simulink model "All_Car_Models"  (R2018b)
settings: Solver=VariableStepAuto  StartTime=0.0  StopTime=10.0  RelTol=1e-3
values from neighbouring files (symbols this model uses):
  a = 1.25    [SetCoefficients_FC.m]
  amplitude = 0.01    [SetCoefficients_FC.m]
  b = 1.4    [SetCoefficients_FC.m]
  c = 1.3    [SetCoefficients_FC.m]
  csc = 600    [SetCoefficients_FC.m]
  cse = 1200    [SetCoefficients_FC.m]
  d = 1.7    [SetCoefficients_FC.m]
  delay = (a+b)/v    [setSpeed.m]
  Fre_r = Fre*2*pi    [setSpeed.m]
  g = 9.81    [SetCoefficients_FC.m]
  HumpHight = 2    [SetCoefficients_FC.m]
  HumpLegnth = 20    [SetCoefficients_FC.m]
  I = 600    [SetCoefficients_FC.m]
  I_phi = 1000    [SetCoefficients_FC.m]
  I_theta = 600    [SetCoefficients_FC.m]
  ks =     [SetCoefficients.m]    (also in SetCoefficients_FC.m = 20000)
  ksSteel = 6.6e9    (= 6600000000)    [SetCoefficients_FC.m]
  ksstiff = 4e5    (= 400000)    [SetCoefficients_FC.m]
  kt =     [SetCoefficients.m]    (also in SetCoefficients_FC.m = 140000)
  m1 = 250    [SetCoefficients.m]    (also in SetCoefficients_FC.m)
  m2 =     [SetCoefficients.m]    (also in SetCoefficients_FC.m = 20)
  mb = 1000    [SetCoefficients_FC.m]
  mbh = mb/2    (= 500)    [SetCoefficients_FC.m]
  v_hump = v    [setSpeed.m]
  x1 = 0.2    [SetCoefficients_FC.m]
  x2 = 0.25    [SetCoefficients_FC.m]
  xt_Lim = 0.1    [SetCoefficients_FC.m]
(part 2 of 2)

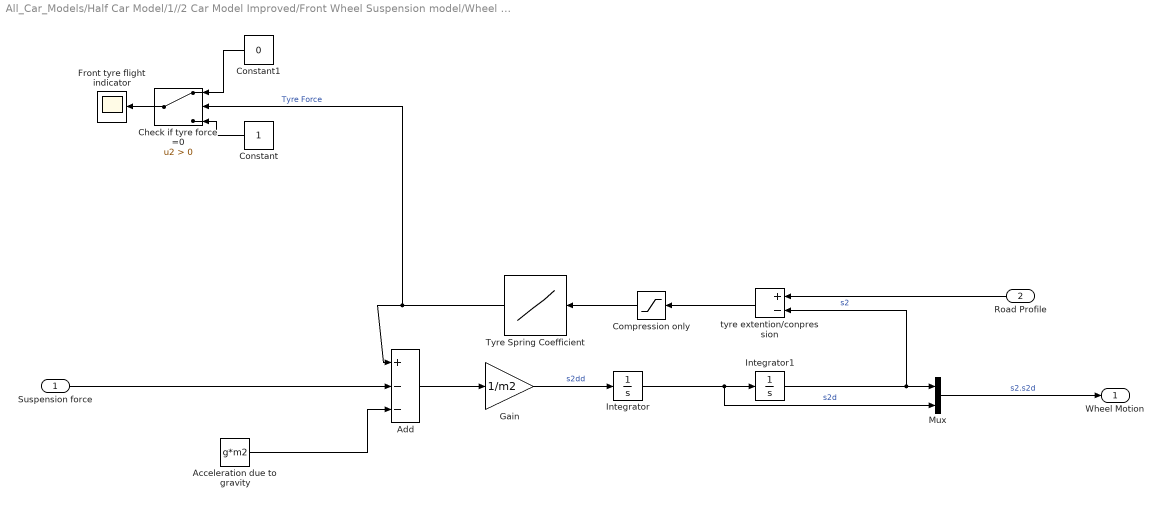
== system All_Car_Models/Half Car Model/1//2 Car Model Improved/Front Wheel Suspension model/Wheel Model ==
  Suspension force : Inport
  Road Profile : Inport  Port=2
  Acceleration due to gravity : Constant  Value=g*m2
  Add : Sum  Inputs=+--
  Check if tyre force =0 : Switch  Criteria=u2 > Threshold
  Compression only : Saturate  UpperLimit=inf  LowerLimit=0
  Constant : Constant
  Constant1 : Constant  Value=0
  Front tyre flight indicator : Scope
  Gain : Gain  Gain=1/m2
  Integrator : Integrator
  Integrator1 : Integrator  InitialCondition=-0.02
  Mux : Mux  Inputs=2
  Tyre Spring Coefficient : Lookup_n-D  NumberOfTableDimensions=1  BreakpointsForDimension1=[0 xt_Lim 2*xt_Lim]  Table=[0 xt_Lim*kt ksSteel*2*xt_Lim]  InternalRulePriority=Speed  RndMeth=Simplest  InputSameDT=on
  tyre extention/conpression : Sum  Inputs=+-
  Wheel Motion : Outport
  wires:
  Integrator1/1 -> Mux/1, tyre extention/conpression/2  "s2"
  Integrator/1 -> Mux/2, Integrator1/1  "s2d"
  Add/1 -> Gain/1
  Tyre Spring Coefficient/1 -> Check if tyre force =0/2, Add/1  "Tyre Force"
  Road Profile/1 -> tyre extention/conpression/1
  Mux/1 -> Wheel Motion/1  "s2.s2d"
  Acceleration due to gravity/1 -> Add/3
  Suspension force/1 -> Add/2
  Gain/1 -> Integrator/1  "s2dd"
  tyre extention/conpression/1 -> Compression only/1
  Compression only/1 -> Tyre Spring Coefficient/1
  Check if tyre force =0/1 -> Front tyre flight indicator/1
  Constant1/1 -> Check if tyre force =0/1
  Constant/1 -> Check if tyre force =0/3

== system All_Car_Models/Half Car Model/1//2 Car Model Improved/Rear Wheel Suspension model/Suspention Model ==
  note: s1.s1d
  note: s2.s2d
  Wheel Motion : Inport
  Body Motion : Inport  Port=2
  " " : Sum  Inputs=+-
  " " : Sum  Inputs=+-
  Add Suspension forces : Sum
  Demux : Demux  Outputs=2
  Demux1 : Demux  Outputs=2
  Suspension Damping Coefficient : Lookup_n-D  NumberOfTableDimensions=1  BreakpointsForDimension1=[-10 0 10]  Table=[-10*cse 0 10*csc]  InternalRulePriority=Speed  RndMeth=Simplest  InputSameDT=on
  Suspension Spring Coefficient : Lookup_n-D  NumberOfTableDimensions=1  BreakpointsForDimension1=([0 x1 x2 2*x2])  Table=([0 ks*x1 ksstiff*(x2-x1)-(ks*x1) ksSteel*x2-(ksstiff*(x2-x1)-(ks*x1))])  InternalRulePriority=Speed  RndMeth=Simplest  InputSameDT=on
  Suspension Force : Outport
  wires:
  Demux1/2 -> " "/2  "s1d"
  " "/1 -> Suspension Spring Coefficient/1  "s1-s2"
  Demux1/1 -> " "/2  "s1"
  Suspension Damping Coefficient/1 -> Add Suspension forces/2
  Suspension Spring Coefficient/1 -> Add Suspension forces/1
  Demux/1 -> " "/1  "s2"
  Demux/2 -> " "/1  "s2d"
  Body Motion/1 -> Demux1/1
  " "/1 -> Suspension Damping Coefficient/1  "s1d-s2d"
  Add Suspension forces/1 -> Suspension Force/1
  Wheel Motion/1 -> Demux/1

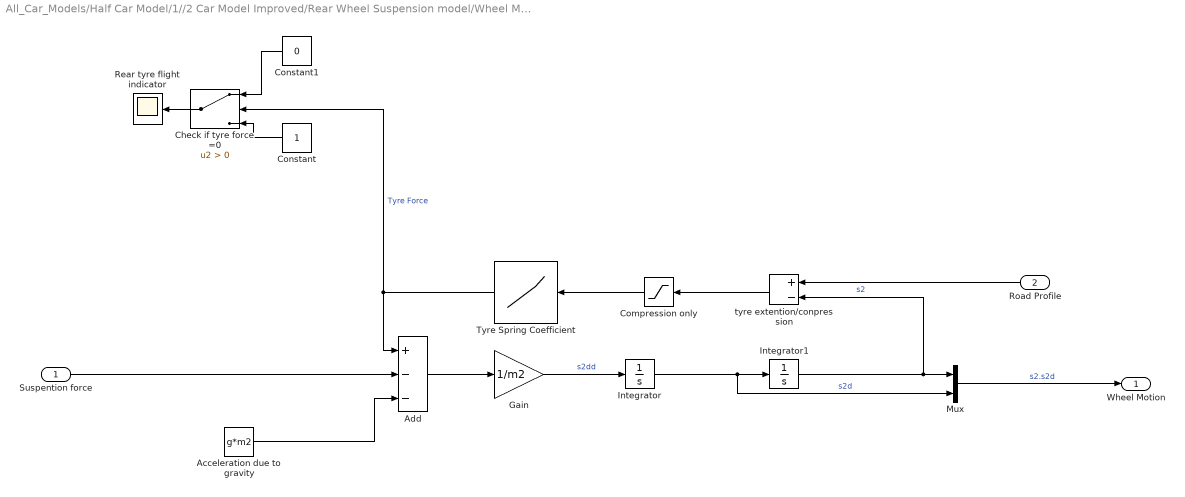
== system All_Car_Models/Half Car Model/1//2 Car Model Improved/Rear Wheel Suspension model/Wheel Model ==
  Suspention force : Inport
  Road Profile : Inport  Port=2
  Acceleration due to gravity : Constant  Value=g*m2
  Add : Sum  Inputs=+--
  Check if tyre force =0 : Switch  Criteria=u2 > Threshold
  Compression only : Saturate  UpperLimit=inf  LowerLimit=0
  Constant : Constant
  Constant1 : Constant  Value=0
  Gain : Gain  Gain=1/m2
  Integrator : Integrator
  Integrator1 : Integrator  InitialCondition=-0.018
  Mux : Mux  Inputs=2
  Rear tyre flight indicator : Scope
  Tyre Spring Coefficient : Lookup_n-D  NumberOfTableDimensions=1  BreakpointsForDimension1=[0 xt_Lim 2*xt_Lim]  Table=[0 xt_Lim*kt ksSteel*2*xt_Lim]  InternalRulePriority=Speed  RndMeth=Simplest  InputSameDT=on
  tyre extention/conpression : Sum  Inputs=+-
  Wheel Motion : Outport
  wires:
  Integrator1/1 -> tyre extention/conpression/2, Mux/1  "s2"
  Integrator/1 -> Mux/2, Integrator1/1  "s2d"
  Add/1 -> Gain/1
  Road Profile/1 -> tyre extention/conpression/1
  Mux/1 -> Wheel Motion/1  "s2.s2d"
  Acceleration due to gravity/1 -> Add/3
  Suspention force/1 -> Add/2
  Gain/1 -> Integrator/1  "s2dd"
  tyre extention/conpression/1 -> Compression only/1
  Constant/1 -> Check if tyre force =0/3
  Check if tyre force =0/1 -> Rear tyre flight indicator/1
  Constant1/1 -> Check if tyre force =0/1
  Compression only/1 -> Tyre Spring Coefficient/1
  Tyre Spring Coefficient/1 -> Add/1, Check if tyre force =0/2  "Tyre Force"
